simulink model "model"  (R2021a)
settings: Solver=VariableStepAuto  StartTime=0.0  StopTime=8  RelTol=1e-3
values from neighbouring files (symbols this model uses):
  etatotKt = 1.8    [script.m]    (also in tf_code.m)
  Jtot = 7.226    [script.m]
  Kb = 2    [script.m]    (also in tf_code.m)
  Kcs = 0.5    [script.m]    (also in tf_code.m)
  Kf = 0.1    [script.m]    (also in tf_code.m)
  Kss = 0.0433    [script.m]    (also in tf_code.m)
  pcwAv0r_itot = 0.6154    [script.m]    (also in tf_code.m)
  r_itot = 0.0615    [script.m]    (also in tf_code.m)
  Ra = 1    [script.m]    (also in tf_code.m)
libraries: simulink x3
settings Model: Creator=ALJAZEERA  LastModifiedBy=ALJAZEERA

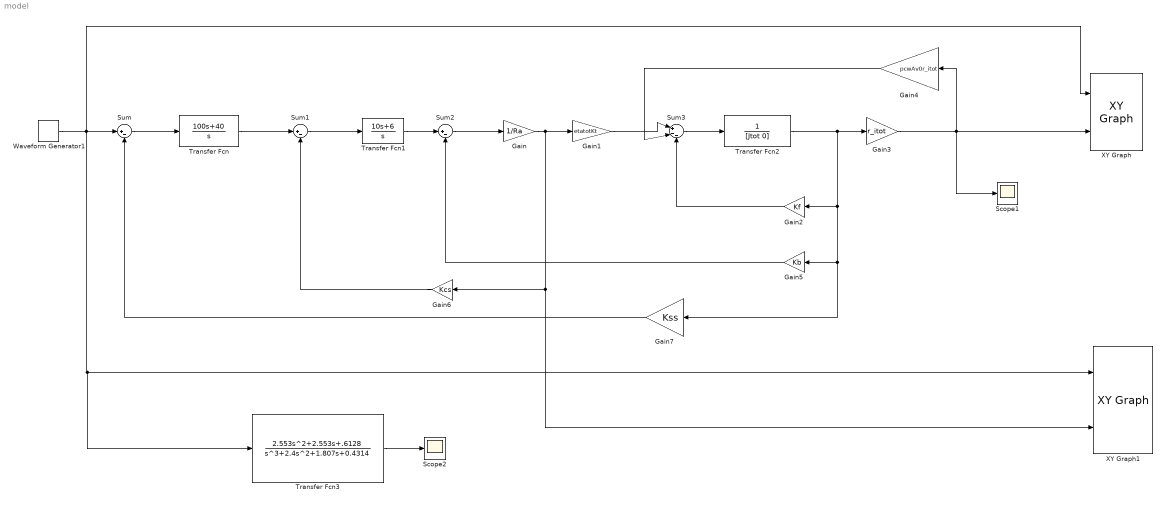
== system model ==
  Gain : Gain  Gain=1/Ra
  Gain1 : Gain  Gain=etatotKt
  Gain2 : Gain  Gain=Kf
  Gain3 : Gain  Gain=r_itot
  Gain4 : Gain  Gain=pcwAv0r_itot
  Gain5 : Gain  Gain=Kb
  Gain6 : Gain  Gain=Kcs
  Gain7 : Gain  Gain=Kss
  Scope1 : Scope
  Scope2 : Scope
  Sum : Sum  Inputs=|+-
  Sum1 : Sum  Inputs=|+-
  Sum2 : Sum  Inputs=|+-
  Sum3 : Sum  Inputs=|+--
  Transfer Fcn : TransferFcn  Description=Gsc(s)  Numerator=[100 40]  Denominator=[1 0]
  Transfer Fcn1 : TransferFcn  Numerator=[10 6]  Denominator=[1 0]
  Transfer Fcn2 : TransferFcn  Denominator=[Jtot 0]
  Transfer Fcn3 : TransferFcn  Numerator=[2.553 2.553 .6128]  Denominator=[1 2.4 1.807 0.4314]
  Waveform Generator1 : simulink/Sources/Waveform Generator  OutMin=[]  OutMax=[]  OutDataTypeStr=double  SelectedSignal=1  Signals=pulse('Amplitude', 1, 'TriggerTime', 1, 'Duration', 2)#sin('Amplitude', 2, 'Frequency', 300, 'Phase', 0)  BlockNames=MultiportSwitch_cbb813dd14414d5#MultiportSwitch_03d94aa116ed4f4  SampleTime=0.1
  XY Graph : simulink/Sinks/XY Graph  xmin=-10  xmax=10  ymin=0  ymax=2  st=-1
  XY Graph1 : simulink/Sinks/XY Graph  xmin=-10  xmax=10  ymin=0  ymax=10  st=-1
  wires:
  Waveform Generator1/1 -> Transfer Fcn3/1, XY Graph1/1, XY Graph/1, Sum/1
  Sum/1 -> Transfer Fcn/1
  Transfer Fcn/1 -> Sum1/1
  Sum1/1 -> Transfer Fcn1/1
  Transfer Fcn1/1 -> Sum2/1
  Sum2/1 -> Gain/1
  Gain/1 -> XY Graph1/2, Gain6/1, Gain1/1
  Gain1/1 -> Sum3/1
  Transfer Fcn2/1 -> Gain7/1, Gain5/1, Gain2/1, Gain3/1
  Sum3/1 -> Transfer Fcn2/1
  Gain4/1 -> Sum3/2
  Gain2/1 -> Sum3/3
  Gain5/1 -> Sum2/2
  Gain6/1 -> Sum1/2
  Gain7/1 -> Sum/2
  Gain3/1 -> Scope1/1, XY Graph/2, Gain4/1
  Transfer Fcn3/1 -> Scope2/1
